simulink model "adacons"  (R2012b)
settings: Solver=ode45  StartTime=0.0  StopTime=600  RelTol=1e-3
settings Model: Creator=Administrator  LastModifiedBy=Administrator

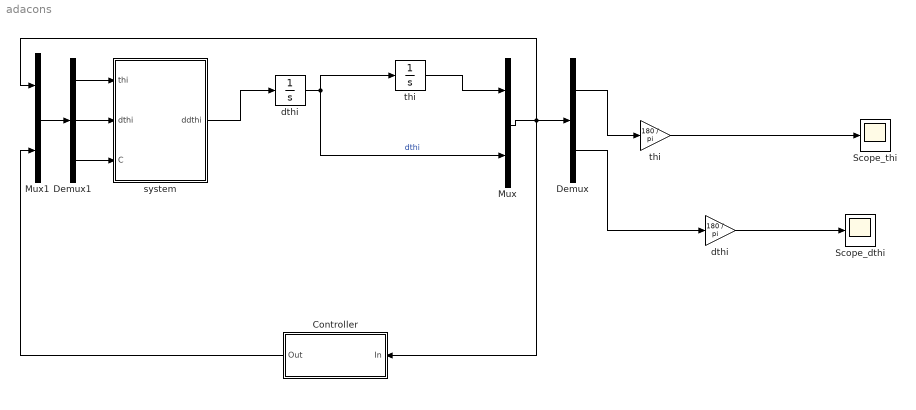
== system adacons ==
  Controller : Subsystem  TreatAsAtomicUnit=on
  Demux : Demux  Outputs=2
  Demux1 : Demux  Outputs=3
  Mux : Mux  Inputs=2
  Mux1 : Mux  Inputs=2
  Scope_dthi : Scope
      settings: SaveName=ScopeData3
  Scope_thi : Scope
      settings: SaveName=ScopeData2
  dthi : Integrator
  "dthi " : Gain  Gain=180 / pi
  system : MATLAB Function  TreatAsAtomicUnit=on
  thi : Integrator  InitialCondition=15 * pi / 180
  "thi " : Gain  Gain=180 / pi
  wires:
  system/1(ddthi) -> dthi/1
  dthi/1 -> Mux/2, thi/1  "dthi"
  thi/1 -> Mux/1
  Mux/1 -> Controller/1(In), Demux/1, Mux1/1
  Mux1/1 -> Demux1/1
  "thi "/1 -> Scope_thi/1
  "dthi "/1 -> Scope_dthi/1
  Controller/1(Out) -> Mux1/2
  Demux/1 -> "thi "/1
  Demux/2 -> "dthi "/1
  Demux1/1 -> system/1(thi)
  Demux1/2 -> system/2(dthi)
  Demux1/3 -> system/3(C)

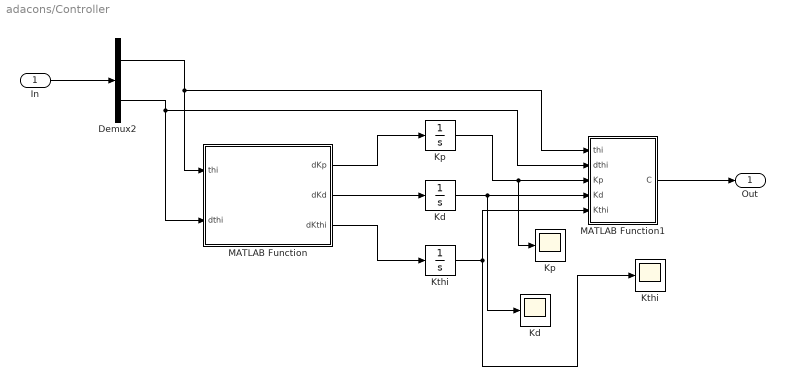
== system adacons/Controller ==
  In : Inport
  Demux2 : Demux  Outputs=2
  Kd : Integrator  InitialCondition=-3218
  "Kd " : Scope
      settings: SaveName=ScopeData6
  Kp : Integrator  InitialCondition=-24720
  "Kp " : Scope
      settings: SaveName=ScopeData4
  Kthi : Integrator  InitialCondition=10
  "Kthi " : Scope
      settings: SaveName=ScopeData5
  MATLAB Function : MATLAB Function  TreatAsAtomicUnit=on
  MATLAB Function1 : MATLAB Function  TreatAsAtomicUnit=on
  Out : Outport
  wires:
  In/1 -> Demux2/1
  Demux2/1 -> MATLAB Function/1(thi), MATLAB Function1/1(thi)
  Demux2/2 -> MATLAB Function1/2(dthi), MATLAB Function/2(dthi)
  MATLAB Function/1(dKp) -> Kp/1
  MATLAB Function/2(dKd) -> Kd/1
  MATLAB Function/3(dKthi) -> Kthi/1
  Kp/1 -> "Kp "/1, MATLAB Function1/3(Kp)
  Kd/1 -> "Kd "/1, MATLAB Function1/4(Kd)
  Kthi/1 -> "Kthi "/1, MATLAB Function1/5(Kthi)
  MATLAB Function1/1(C) -> Out/1

== matlab function adacons/Controller/MATLAB Function ==
  data: thi input; dKp output; dthi input; dKd output; dKthi output
function [dKp, dKd, dKthi] = fcn(thi, dthi)
wn = 10;
ksi = 0.707;
gama1 = -4;
gama2 = -10;
P = [(ksi / wn) + ((wn ^ 2 + 1) / (4 * ksi))     1 / (2 * wn ^ 2); ...
    1 / (2 * wn ^ 2)                             (wn ^ 2 + 1) / (4 * ksi * wn ^ 3)];
T = [0 0;thi dthi];
X = [thi;dthi];
A = gama1 * T' * P * X;
dKp = A(1);
dKd = A(2);
s = thi / (2 * wn ^ 2) + dthi * (wn ^ 2 + 1) / (4 * ksi * wn ^ 3);
dKthi = -gama2 * abs(s);
end

== matlab function adacons/system ==
  data: thi input; dthi input; C input; ddthi output
function ddthi  = fcn(thi,dthi,C)
Mp = 200;
L = 1;
Jp = 27.6;
g = 9.8;

beta = Jp / (Mp * L) + L;
gama = L * Mp * g;
A43 = gama / Jp - (L * gama) / (Jp * beta);
B4 = (L / beta - 1) / Jp;

f4 = 3;

ddthi = A43 * thi + B4 * C + f4;

== matlab function adacons/Controller/MATLAB Function1 ==
  data: thi input; dthi input; Kp input; C output; Kd input; Kthi input
function C = fcn(thi, dthi, Kp, Kd, Kthi)
wn = 10;
ksi = 0.707;
s = thi / (2 * wn ^ 2) + dthi * (wn ^ 2 + 1) / (4 * ksi * wn ^ 3);
u = Kthi * sign(s);
C = -Kp * thi - Kd * dthi + u;
end
